simulink model "IMU_Reader"  (R2025b)
settings: Solver=VariableStepAuto  StartTime=0.0  StopTime=inf  RelTol=1e-3
InitFcn:
  | Ts=0.1;
libraries: instrumentseriallib x2
settings Model: Creator=amind  LastModifiedBy=amind
settings SolverCC: AlgebraicLoopSolver=TrustRegion
settings OptimizationCC: ReuseModelBlockBuffer=off
settings DebuggingCC: UnconnectedInputMsg=warning  UnconnectedOutputMsg=warning  UnconnectedLineMsg=warning
settings ModelReferenceCC: EnableRefExpFcnMdlSchedulingChecks=on
settings RTWCC: GPUComputeCapability=3.5

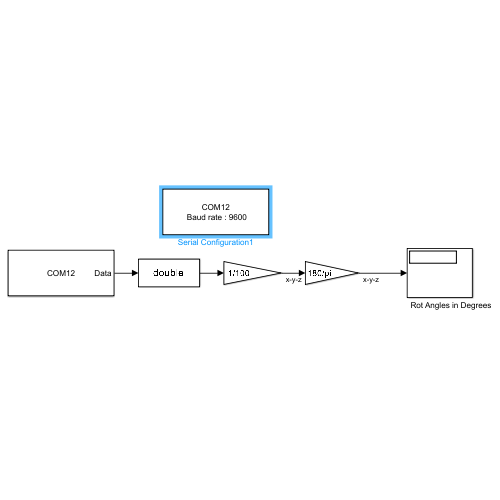
[thumbnail: Simulink's stored preview of the top-level diagram]
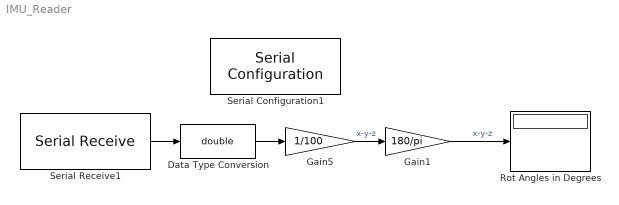
== system IMU_Reader ==
  "          Rot Angles in Degrees" : Display
  Data Type Conversion : DataTypeConversion  OutDataTypeStr=double  SaturateOnIntegerOverflow=off  RndMeth=Floor
  Gain1 : Gain  Gain=180/pi
  Gain5 : Gain  Gain=1/100
  Serial Configuration1 : instrumentseriallib/Serial Configuration  Priority=-200000  PortSel=COM12  Port=COM12  ComPort=COM12  BaudRate=9600  DataBits=8  Parity=none  StopBits=1  ByteOrder=little-endian  FlowControl=none  Timeout=60  SimulateUsing=Interpreted execution  BlockInModel=on  aMode=1
  Serial Receive1 : instrumentseriallib/Serial Receive  Priority=1  PortSel=COM12  Port=COM12  ComPort=COM12  DataType=int16  SaveDataType=uint8  ToggleHeader=off  Header=[]  ToggleDataSize=on  DataSize=[3 1]  ToggleTerminator=off  Terminator=<none>  CustomTerminator=[]  InputFormat=Column major  EnableBlockingMode=on  ActionDataUnavailable=Output last received value  ActionWhenDataUnavailable=Output last received value  CustomValue=0  SampleTime=Ts  SimulateUsing=Interpreted execution  BlockInModel=on  aMode=1  LibraryInUse=instrumentlib
  wires:
  Serial Receive1/1 -> Data Type Conversion/1
  Data Type Conversion/1 -> Gain5/1
  Gain5/1 -> Gain1/1  "x-y-z"
  Gain1/1 -> "          Rot Angles in Degrees"/1  "x-y-z"
